simulink model "Controller_2_CalcSTD"  (Simulink 7.5)
settings: Solver=ode45  StartTime=0.0  StopTime=10.0  RelTol=1e-3
undefined symbols (not defined in the file): ctrller
settings Model: Creator=sriddle  LastModifiedBy=sriddle

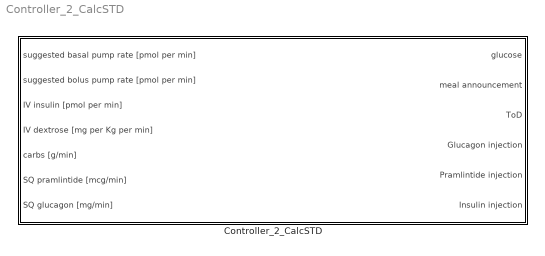
== system Controller_2_CalcSTD ==
  Controller_2_CalcSTD : Subsystem

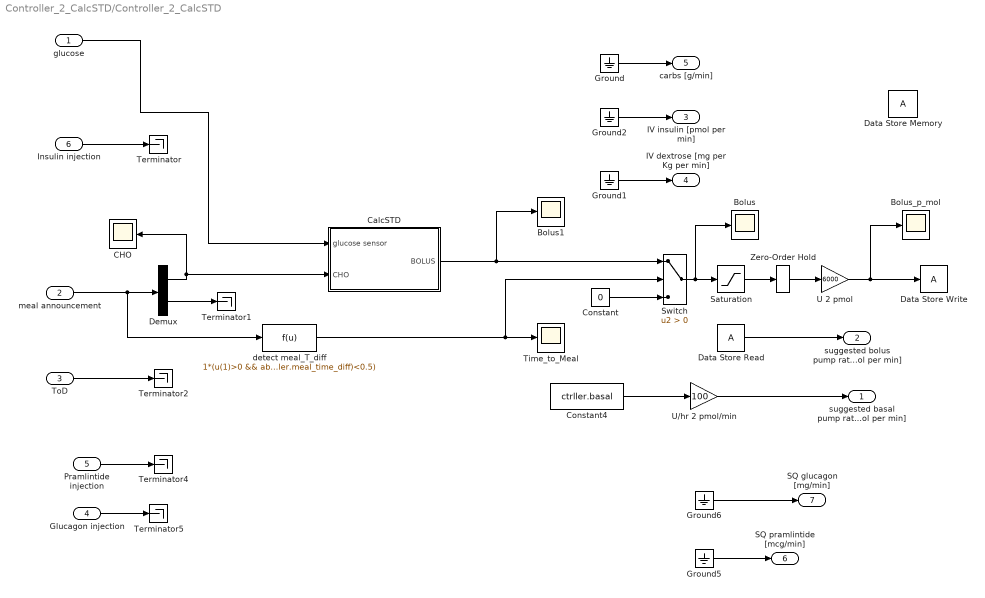
== system Controller_2_CalcSTD/Controller_2_CalcSTD ==
  glucose : Inport  OutDataType=sfix(16)  OutScaling=2^0
  meal announcement : Inport  Port=2  OutDataType=sfix(16)  OutScaling=2^0
  ToD : Inport  Port=3  OutDataType=sfix(16)  OutScaling=2^0
  Glucagon injection : Inport  Port=4
  Pramlintide injection : Inport  Port=5
  Insulin injection : Inport  Port=6  OutDataType=sfix(16)  OutScaling=2^0
  Bolus : Scope
      settings: YMin=0  YMax=3000  SaveName=ScopeData2
  Bolus1 : Scope
      settings: SaveName=ScopeData10
  Bolus_p_mol : Scope
      settings: YMin=0  YMax=60000  SaveName=ScopeData5
  CHO : Scope
      settings: YMin=0  YMax=0.01
  CalcSTD : Subsystem
  Constant : Constant  Value=0  OutDataType=sfix(16)  OutScaling=2^0
  Constant4 : Constant  Value=ctrller.basal  OutDataType=sfix(16)  OutScaling=2^0
  Data Store Memory : DataStoreMemory  DataStoreName=A  ReadBeforeWriteMsg=warning  WriteAfterWriteMsg=warning  WriteAfterReadMsg=warning  OutDataType=fixdt(1, 16)  OutScaling=2^0
  Data Store Read : DataStoreRead  DataStoreName=A  SampleTime=0
  Data Store Write : DataStoreWrite  DataStoreName=A  SampleTime=-1
  Demux : Demux  Outputs=2
  Ground{,1..2,5..6} (5 alike) : Ground
  Saturation : Saturate  UpperLimit=100  LowerLimit=0  OutDataType=fixdt(1, 16)  OutScaling=2^0
  Switch : Switch  Criteria=u2 > Threshold  OutDataType=sfix(16)  OutScaling=2^0
  Terminator{,1..2,4..5} (5 alike) : Terminator
  Time_to_Meal : Scope
      settings: SaveName=ScopeData3
  U 2 pmol : Gain  Gain=6000  ParameterDataType=sfix(16)  ParameterScaling=2^0  OutDataType=sfix(16)  OutScaling=2^0
  U/hr 2 pmol/min : Gain  Gain=100  ParameterDataType=sfix(16)  ParameterScaling=2^0  OutDataType=sfix(16)  OutScaling=2^0
  Zero-Order Hold : ZeroOrderHold
  detect meal_T_diff : Fcn  Expr=1*(u(1)>0 && abs(u(2)+ctrller.meal_time_diff)<0.5)
  suggested basal pump rate [pmol per min] : Outport  OutDataType=sfix(16)  OutScaling=2^0
  suggested bolus pump rate [pmol per min] : Outport  Port=2  OutDataType=sfix(16)  OutScaling=2^0
  IV insulin [pmol per min] : Outport  Port=3  OutDataType=sfix(16)  OutScaling=2^0
  IV dextrose [mg per Kg per min] : Outport  Port=4  OutDataType=sfix(16)  OutScaling=2^0
  carbs [g/min] : Outport  Port=5  OutDataType=sfix(16)  OutScaling=2^0
  SQ pramlintide [mcg/min] : Outport  Port=6
  SQ glucagon [mg/min] : Outport  Port=7
  wires:
  Ground1/1 -> IV dextrose [mg per Kg per min]/1
  Ground2/1 -> IV insulin [pmol per min]/1
  Ground/1 -> carbs [g/min]/1
  Data Store Read/1 -> suggested bolus pump rate [pmol per min]/1
  U 2 pmol/1 -> Data Store Write/1, Bolus_p_mol/1
  U/hr 2 pmol/min/1 -> suggested basal pump rate [pmol per min]/1
  Zero-Order Hold/1 -> U 2 pmol/1
  Constant4/1 -> U/hr 2 pmol/min/1
  Constant/1 -> Switch/3
  detect meal_T_diff/1 -> Switch/2, Time_to_Meal/1
  ToD/1 -> Terminator2/1
  Insulin injection/1 -> Terminator/1
  glucose/1 -> CalcSTD/1(glucose sensor)
  Demux/1 -> CHO/1, CalcSTD/2(CHO)
  meal announcement/1 -> Demux/1, detect meal_T_diff/1
  Saturation/1 -> Zero-Order Hold/1
  Switch/1 -> Saturation/1, Bolus/1
  Demux/2 -> Terminator1/1
  CalcSTD/1(BOLUS) -> Switch/1, Bolus1/1
  Pramlintide injection/1 -> Terminator4/1
  Glucagon injection/1 -> Terminator5/1
  Ground6/1 -> SQ glucagon [mg/min]/1
  Ground5/1 -> SQ pramlintide [mcg/min]/1

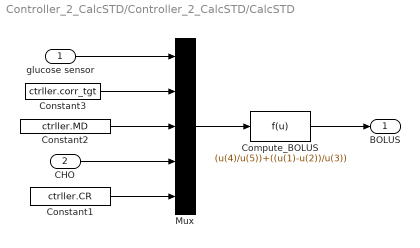
== system Controller_2_CalcSTD/Controller_2_CalcSTD/CalcSTD ==
  glucose sensor : Inport  OutDataType=fixdt(1, 16)  OutScaling=2^0
  CHO : Inport  Port=2  OutDataType=fixdt(1, 16)  OutScaling=2^0
  Compute_BOLUS : Fcn  Expr=(u(4)/u(5))+((u(1)-u(2))/u(3))
  Constant1 : Constant  Value=ctrller.CR  OutDataType=sfix(16)  OutScaling=2^0
  Constant2 : Constant  Value=ctrller.MD  OutDataType=sfix(16)  OutScaling=2^0
  Constant3 : Constant  Value=ctrller.corr_tgt  OutDataType=sfix(16)  OutScaling=2^0
  Mux : Mux  Inputs=5
  BOLUS : Outport  OutDataType=fixdt(1, 16)  OutScaling=2^0
  wires:
  glucose sensor/1 -> Mux/1
  Constant3/1 -> Mux/2
  Constant2/1 -> Mux/3
  CHO/1 -> Mux/4
  Constant1/1 -> Mux/5
  Mux/1 -> Compute_BOLUS/1
  Compute_BOLUS/1 -> BOLUS/1
